simulink model "uavsim_trim"  (R2015a)
settings: Solver=ode45  StartTime=0.0  StopTime=10.0  RelTol=1e-3
undefined symbols (not defined in the file or in its folder): forces_moments, UAV
settings Model: Creator=User  LastModifiedBy=User

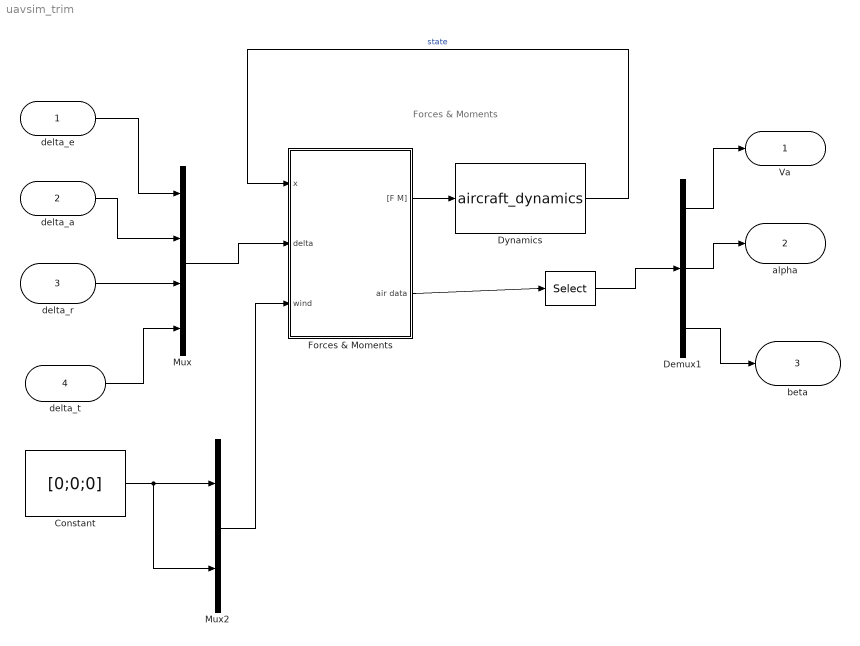
== system uavsim_trim ==
  note: Forces & Moments
  delta_e : Inport
  delta_a : Inport  Port=2
  delta_r : Inport  Port=3
  delta_t : Inport  Port=4
  " " : Selector  InputPortWidth=6  Indices=[1 2 3]
  Constant : Constant  Value=[0;0;0]
  Demux1 : Demux  Outputs=3
  Dynamics : S-Function  FunctionName=aircraft_dynamics  Parameters=UAV
  Forces & Moments : Subsystem
  Mux : Mux
  Mux2 : Mux  Inputs=2
  Va : Outport
  alpha : Outport  Port=2
  beta : Outport  Port=3
  wires:
  delta_e/1 -> Mux/1
  delta_a/1 -> Mux/2
  delta_r/1 -> Mux/3
  delta_t/1 -> Mux/4
  Mux/1 -> Forces & Moments/2(delta)
  Constant/1 -> Mux2/2, Mux2/1
  Mux2/1 -> Forces & Moments/3(wind)
  Forces & Moments/1("[F M]") -> Dynamics/1
  Dynamics/1 -> Forces & Moments/1(x)  "state"
  Forces & Moments/2(air data) -> " "/1
  " "/1 -> Demux1/1
  Demux1/1 -> Va/1
  Demux1/2 -> alpha/1
  Demux1/3 -> beta/1

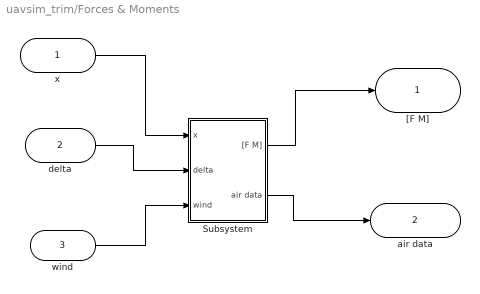
== system uavsim_trim/Forces & Moments ==
  x : Inport
  delta : Inport  Port=2
  wind : Inport  Port=3
  Subsystem : Subsystem
  "[F M]" : Outport
  air data : Outport  Port=2
  wires:
  Subsystem/1("[F M]") -> "[F M]"/1
  wind/1 -> Subsystem/3(wind)
  x/1 -> Subsystem/1(x)
  delta/1 -> Subsystem/2(delta)
  Subsystem/2(air data) -> air data/1

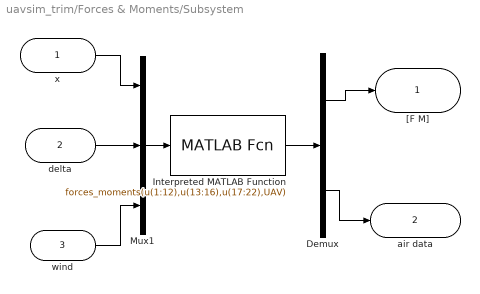
== system uavsim_trim/Forces & Moments/Subsystem ==
  x : Inport
  delta : Inport  Port=2
  wind : Inport  Port=3
  Demux : Demux  Outputs=[6;6]
  Interpreted MATLAB Function : MATLABFcn  MATLABFcn=forces_moments(u(1:12),u(13:16),u(17:22),UAV)  OutputDimensions=12
  Mux1 : Mux  Inputs=3
  "[F M]" : Outport
  air data : Outport  Port=2
  wires:
  delta/1 -> Mux1/2
  wind/1 -> Mux1/3
  Interpreted MATLAB Function/1 -> Demux/1
  Demux/1 -> "[F M]"/1
  x/1 -> Mux1/1
  Demux/2 -> air data/1
  Mux1/1 -> Interpreted MATLAB Function/1
